simulink model "Led"  (R2018a)
settings: Solver=FixedStepDiscrete  StartTime=0.0  StopTime=10.0  RelTol=1e-3
libraries: simulink x1
settings Model: Creator=Ahmed-Yehia  LastModifiedBy=Ahmed-Yehia
settings OptimizationCC: DefaultParameterBehavior=Inlined  EnhancedBackFolding=on  PassReuseOutputArgsAs=Individual arguments  OptimizeBlockOrder=speed  DifferentSizesBufferReuse=on  OptimizationCustomize=off
settings DebuggingCC: UnderspecifiedInitializationDetection=Classic  MergeDetectMultiDrivingBlocksExec=none  ParameterTunabilityLossMsg=error
settings ModelReferenceCC: PropagateSignalLabelsOutOfModel=off
settings SFSimCC: MATLABDynamicMemAlloc=off
settings RTWCC: SystemTargetFile=ert.tlc  GenCodeOnly=on  TemplateMakefile=ert_default_tmf  GenerateReport=on  IncludeHyperlinkInReport=on  LaunchReport=on  GenerateTraceInfo=on  GenerateTraceReport=on  GenerateTraceReportSl=on  GenerateTraceReportSf=on  GenerateTraceReportEml=on
settings CodeAppCC: ForceParamTrailComments=on  IgnoreCustomStorageClasses=off  OperatorAnnotations=on  SimulinkDataObjDesc=on  SFDataObjDesc=on  InsertBlockDesc=on
settings ERTTargetCC: TargetLangStandard=C99 (ISO)  GenerateSampleERTMain=on  InlinedParameterPlacement=NonHierarchical  ERTCustomFileTemplate=example_file_process.tlc

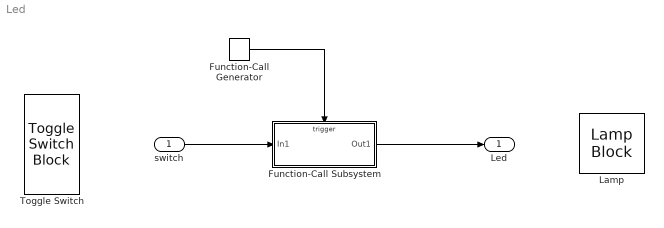
== system Led ==
  switch : Inport
  Function-Call Generator : simulink/Ports & Subsystems/Function-Call Generator  sample_time=0.005  numberOfIterations=1
  Function-Call Subsystem : Subsystem  TreatAsAtomicUnit=on
  Lamp : LampBlock  WebBlockId=13
  Toggle Switch : ToggleSwitchBlock  WebBlockId=9
      settings: Values={{'Off', 'On'}, [0 1]}
  Led : Outport
  wires:
  Function-Call Generator/1 -> Function-Call Subsystem/Trigger
  switch/1 -> Function-Call Subsystem/1(In1)
  Function-Call Subsystem/1(Out1) -> Led/1

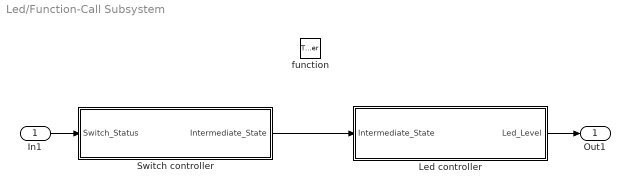
== system Led/Function-Call Subsystem ==
  In1 : Inport
  function : TriggerPort  TriggerType=function-call  VariantControl=Variant
  Led controller : Stateflow chart  TreatAsAtomicUnit=on
  Switch controller : Stateflow chart  TreatAsAtomicUnit=on
  Out1 : Outport
  wires:
  In1/1 -> Switch controller/1(Switch_Status)
  Switch controller/1(Intermediate_State) -> Led controller/1(Intermediate_State)
  Led controller/1(Led_Level) -> Out1/1

== stateflow chart Led/Function-Call Subsystem/Led controller ==
  (default) -> (junction 15) : /* check the intermediate status */
  (junction 15) -> (junction 16) [order 1] : [Intermediate_State == 1]
  (junction 15) -> (junction 19) [order 2]
  (junction 16) -> (junction 17) : {Led_Level = 1;}
  (junction 17) -> (junction 18)
  (junction 18) -> (junction 22)
  (junction 19) -> (junction 20) [order 1] : [Intermediate_State == 0]
  (junction 19) -> (junction 23) [order 2]
  (junction 20) -> (junction 21) : {Led_Level = 0;}
  (junction 21) -> (junction 22)
  (junction 22) -> (junction 24)
  (junction 24) -> (junction 23)
  (junction 23) -> (junction 25)
  data: Intermediate_State input double; Led_Level output double

== stateflow chart Led/Function-Call Subsystem/Switch controller ==
  (default) -> (junction 15) : /* check the switch status */
  (junction 15) -> (junction 16) [order 1] : [Switch_Status == 1]
  (junction 15) -> (junction 19) [order 2]
  (junction 16) -> (junction 17) : {Intermediate_State = 1;}
  (junction 17) -> (junction 18)
  (junction 18) -> (junction 22)
  (junction 19) -> (junction 20) [order 1] : [Switch_Status == 0]
  (junction 19) -> (junction 23) [order 2]
  (junction 20) -> (junction 21) : {Intermediate_State = 0;}
  (junction 21) -> (junction 22)
  (junction 22) -> (junction 24)
  (junction 24) -> (junction 23)
  (junction 23) -> (junction 25)
  data: Intermediate_State output double; Switch_Status input double
